simulink model "zadanie2mdl"  (Simulink 7.2)
settings: Solver=ode4  SolverMode=SingleTasking  StartTime=0.0  StopTime=10.0  FixedStep=1e-2  RelTol=1e-3
values from neighbouring files (symbols this model uses):
  A = [-5, 1; -1, -5]    [zadanie2.m]    (also in zadanie3.m = [0, 0; 0, -1])
  Ap = expm(h*A)    [zadanie2.m]    (also in zadanie3.m)
  B = [1; 0]    [zadanie2.m]    (also in zadanie3.m = [1; 1])
  Bp = double( int(expm(s*A)*B,s,0,h))    [zadanie2.m]    (also in zadanie3.m)
  C = [0, 1]    [zadanie2.m]    (also in zadanie3.m)
  Cp = C    [zadanie2.m]    (also in zadanie3.m)
  h = h*h    [zadanie2.m]    (also in zadanie3.m)
settings Model: Creator=Jacek  LastModifiedBy=lab111
settings DataIOCC: LimitDataPoints=off  SignalLoggingName=sigsOut
settings DebuggingCC: SaveWithParameterizedLinksMsg=none  SignalResolutionControl=TryResolveAllWithWarning  SolverPrmCheckMsg=none  MultiTaskDSMMsg=warning  MultiTaskCondExecSysMsg=none  StrictBusMsg=None
settings HardwareCC: TargetUnknown=on
settings RTWCC: IncludeERTFirstTime=on

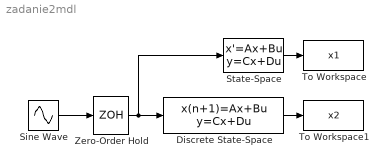
== system zadanie2mdl ==
  Discrete State-Space : DiscreteStateSpace  A=Ap  B=Bp  C=Cp  D=0  SampleTime=h
  Sine Wave : Sin  SampleTime=0
  State-Space : StateSpace  A=A  B=B  C=C  D=0
  To Workspace : ToWorkspace  VariableName=x1  SampleTime=-1  SaveFormat=Array
  To Workspace1 : ToWorkspace  VariableName=x2  SampleTime=-1  SaveFormat=Array
  Zero-Order Hold : ZeroOrderHold  SampleTime=h
  wires:
  Sine Wave/1 -> Zero-Order Hold/1
  State-Space/1 -> To Workspace/1
  Discrete State-Space/1 -> To Workspace1/1
  Zero-Order Hold/1 -> Discrete State-Space/1, State-Space/1
